simulink library "CalculationGallon"  (R2017b)
settings: Solver=VariableStepAuto  StartTime=0.0  StopTime=10.0  RelTol=1e-3
undefined symbols (not defined in the file): DiscIntNeverNeededParam, Engine
libraries: simulink x3
settings Model: Creator=Lyu19  LastModifiedBy=Lyu19

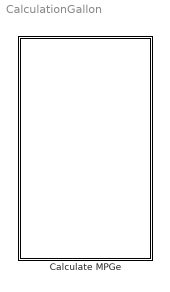
== system CalculationGallon ==
  Calculate MPGe : Subsystem

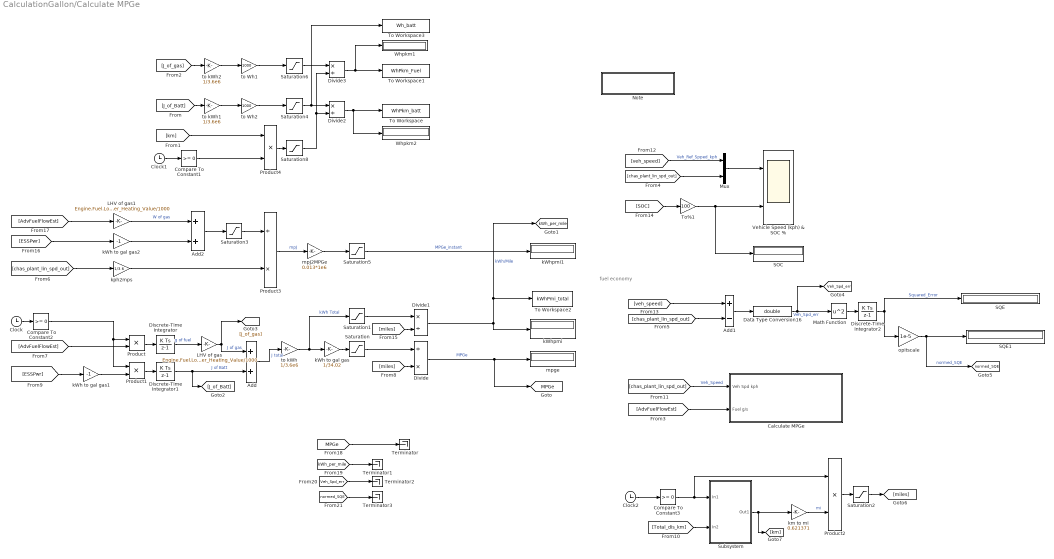
== system CalculationGallon/Calculate MPGe ==
  note: fuel economy
  Add : Sum
  Add1 : Sum  Inputs=+-
  Add2 : Sum
  Calculate MPGe : Subsystem
  Clock : Clock
  Clock1 : Clock
  Clock2 : Clock
  Compare To Constant1 : simulink/Logic and Bit Operations/Compare To Constant  relop=>=  const=0  OutDataTypeStr=boolean
  Compare To Constant2 : simulink/Logic and Bit Operations/Compare To Constant  relop=>=  const=0  OutDataTypeStr=boolean
  Compare To Constant3 : simulink/Logic and Bit Operations/Compare To Constant  relop=>=  const=0  OutDataTypeStr=boolean
  Data Type Conversion16 : DataTypeConversion  OutDataTypeStr=double
  Discrete-Time Integrator : DiscreteIntegrator  SampleTime=-1  ICPrevOutput=DiscIntNeverNeededParam  ICPrevScaledInput=DiscIntNeverNeededParam
  Discrete-Time Integrator1 : DiscreteIntegrator  SampleTime=-1  ICPrevOutput=DiscIntNeverNeededParam  ICPrevScaledInput=DiscIntNeverNeededParam
  Discrete-Time Integrator2 : DiscreteIntegrator  SampleTime=-1  ICPrevOutput=DiscIntNeverNeededParam  ICPrevScaledInput=DiscIntNeverNeededParam
  Divide : Product  Inputs=/*
  Divide1 : Product  Inputs=*/
  Divide2 : Product  Inputs=*/
  Divide3 : Product  Inputs=*/
  LHV of gas : Gain  Gain=Engine.Fuel.Lower_Heating_Value/1000
  LHV of gas1 : Gain  Gain=Engine.Fuel.Lower_Heating_Value/1000
  Math Function : Math  Operator=square  SaturateOnIntegerOverflow=on
  Mux : Mux  Inputs=2
  Note : Subsystem
  Product{,1..2,4} (4 alike) : Product
  Product3 : Product  Inputs=/*
  SOC : Display
  SQE : Display
  SQE1 : Display
  Saturation{,1..4,6,8} (7 alike) : Saturate  UpperLimit=inf  LowerLimit=1e-6
  Saturation5 : Saturate  UpperLimit=80  LowerLimit=1e-6
  Subsystem : Subsystem
  Terminator{,1..3} (4 alike) : Terminator
  To Workspace : ToWorkspace  VariableName=WhPkm_batt  SampleTime=-1
  To Workspace1 : ToWorkspace  VariableName=WhPkm_Fuel  SampleTime=-1
  To Workspace2 : ToWorkspace  VariableName=kWhPmi_total  SampleTime=-1
  To Workspace3 : ToWorkspace  VariableName=Wh_batt  SampleTime=-1
  To%1 : Gain  Gain=100
  Vehicle Speed (kph) & SOC % : Scope  NumInputPorts=2
  Whpkm1 : Display
  Whpkm2 : Display
  kWh to gal gas : Gain  Gain=1/34.02
  kWh to gal gas1 : Gain  Gain=-1
  kWh to gal gas2 : Gain  Gain=-1
  kWhpmi : Display
  kWhpmi1 : Display
  km to mi : Gain  Gain=0.621371
  kph2mps : Gain  Gain=1/3.6
  mpJ2MPGe : Gain  Gain=0.013*1e6
  mpge : Display
  opitscale : Gain  Gain=1e-5
  to Wh1 : Gain  Gain=1000
  to Wh2 : Gain  Gain=1000
  to kWh : Gain  Gain=1/3.6e6
  to kWh1 : Gain  Gain=1/3.6e6
  to kWh2 : Gain  Gain=1/3.6e6
  tag scope: MPGe=global, Veh_Spd_err=global, kWh_per_mile=global, normed_SQE=global
  wires:
  Discrete-Time Integrator/1 -> LHV of gas/1  "g of fuel"
  LHV of gas/1 -> Add/1, [J_of_gas]  "J of gas"
  Discrete-Time Integrator1/1 -> Add/2, [J_of_Batt]  "J of Batt"
  Add/1 -> to kWh/1  "J total"
  to kWh/1 -> kWh to gal gas/1, Saturation1/1  "kWh Total"
  km to mi/1 -> Product2/2  "mi"
  kWh to gal gas/1 -> Saturation/1
  Divide/1 -> [MPGe], mpge/1  "MPGe"
  [AdvFuelFlowEst] -> Product/2
  [Total_dis_km] -> Subsystem/2(In2)
  Saturation/1 -> Divide/1
  Saturation1/1 -> Divide1/1
  Divide1/1 -> kWhpmi/1, [kWh_per_mile], To Workspace2/1  "kWh/Mile"
  [veh_speed] -> Mux/1  "Veh_Ref_Spped_kph"
  Mux/1 -> Vehicle Speed (kph) & SOC %/1
  [chas_plant_lin_spd_out] -> Calculate MPGe/1(Veh Spd kph)  "Veh_Speed"
  Discrete-Time Integrator2/1 -> opitscale/1, SQE/1  "Squared_Error"
  Data Type Conversion16/1 -> Math Function/1, [Veh_Spd_err]  "Veh_Spd_err"
  opitscale/1 -> [normed_SQE], SQE1/1  "normed_SQE"
  Math Function/1 -> Discrete-Time Integrator2/1
  Saturation2/1 -> [miles]
  Subsystem/1(Out1) -> km to mi/1, [km]
  Clock/1 -> Compare To Constant2/1
  Product/1 -> Discrete-Time Integrator/1
  Compare To Constant2/1 -> Product1/1, Product/1
  Product1/1 -> Discrete-Time Integrator1/1
  Add1/1 -> Data Type Conversion16/1
  Product2/1 -> Saturation2/1
  LHV of gas1/1 -> Add2/1  "W of gas"
  Product3/1 -> mpJ2MPGe/1  "mpJ"
  mpJ2MPGe/1 -> Saturation5/1
  Add2/1 -> Saturation3/1
  Saturation5/1 -> kWhpmi1/1  "MPGe_instant"
  kph2mps/1 -> Product3/2
  Saturation3/1 -> Product3/1
  [J_of_Batt] -> to kWh1/1
  to kWh1/1 -> to Wh2/1
  to Wh2/1 -> Saturation4/1
  Saturation4/1 -> To Workspace3/1, Divide2/1
  Divide2/1 -> Whpkm2/1, To Workspace/1
  [J_of_gas] -> to kWh2/1
  to kWh2/1 -> to Wh1/1
  to Wh1/1 -> Saturation6/1
  Saturation6/1 -> Divide3/1
  Divide3/1 -> Whpkm1/1, To Workspace1/1
  [km] -> Product4/1
  Product4/1 -> Saturation8/1
  Saturation8/1 -> Divide3/2, Divide2/2
  [ESSPwr] -> kWh to gal gas1/1
  kWh to gal gas1/1 -> Product1/2
  Clock1/1 -> Compare To Constant1/1
  Compare To Constant1/1 -> Product4/2
  [AdvFuelFlowEst] -> Calculate MPGe/2(Fuel g/s)
  [chas_plant_lin_spd_out] -> Add1/2
  [chas_plant_lin_spd_out] -> Mux/2
  [chas_plant_lin_spd_out] -> kph2mps/1
  [veh_speed] -> Add1/1
  [SOC] -> To%1/1
  To%1/1 -> SOC/1, Vehicle Speed (kph) & SOC %/2
  Clock2/1 -> Compare To Constant3/1
  Compare To Constant3/1 -> Product2/1, Subsystem/1(In1)
  [miles] -> Divide/2
  [miles] -> Divide1/2
  [ESSPwr] -> kWh to gal gas2/1
  kWh to gal gas2/1 -> Add2/2
  [AdvFuelFlowEst] -> LHV of gas1/1
  [MPGe] -> Terminator/1
  [kWh_per_mile] -> Terminator1/1
  [Veh_Spd_err] -> Terminator2/1
  [normed_SQE] -> Terminator3/1

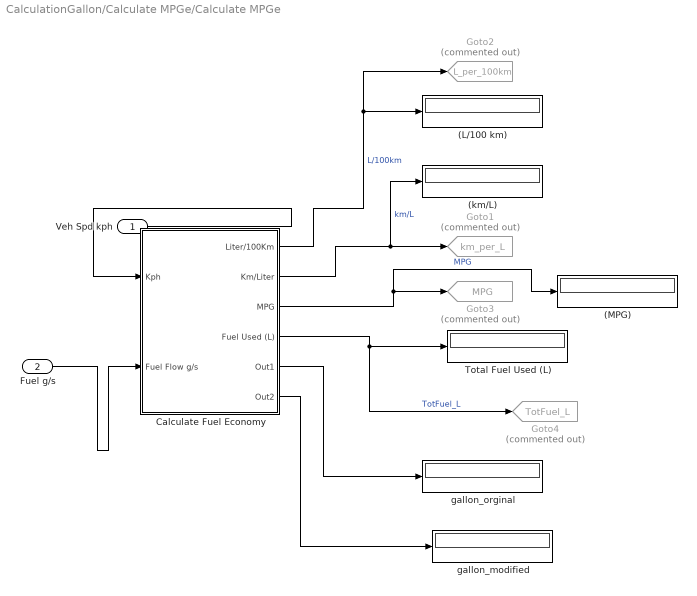
== system CalculationGallon/Calculate MPGe/Calculate MPGe ==
  Veh Spd kph : Inport
  Fuel g/s : Inport  Port=2
  (L/100 km) : Display
  (MPG) : Display
  (km/L) : Display
  Calculate Fuel Economy : Subsystem
  Goto1 : Goto  Commented=on  GotoTag=km_per_L  TagVisibility=global
  Goto2 : Goto  Commented=on  GotoTag=L_per_100km  TagVisibility=global
  Goto3 : Goto  Commented=on  GotoTag=MPG  TagVisibility=global
  Goto4 : Goto  Commented=on  GotoTag=TotFuel_L  TagVisibility=global
  Total Fuel Used (L) : Display
  gallon_modified : Display
  gallon_orginal : Display
  wires:
  Fuel g/s/1 -> Calculate Fuel Economy/2(Fuel Flow g/s)
  Calculate Fuel Economy/1(Liter/100Km) -> Goto2/1, (L/100 km)/1  "L/100km"
  Calculate Fuel Economy/3(MPG) -> Goto3/1, (MPG)/1  "MPG"
  Calculate Fuel Economy/4(Fuel Used (L)) -> Goto4/1, Total Fuel Used (L)/1  "TotFuel_L"
  Calculate Fuel Economy/2(Km/Liter) -> (km/L)/1, Goto1/1  "km/L"
  Veh Spd kph/1 -> Calculate Fuel Economy/1(Kph)
  Calculate Fuel Economy/5(Out1) -> gallon_orginal/1
  Calculate Fuel Economy/6(Out2) -> gallon_modified/1

== system CalculationGallon/Calculate MPGe/Note ==
  note: Note that this is calculating the
      | instantaneous MPGe over time
      | (includes fuel and battery energy used).
      |
      | You should also look at the SOC
      | or energy of the Battery at the end
      | of the cycle, and see what the delta
      | is between the start/end.  If more/less
      | energy is in the Battery at the end, you
      | should determine how you want to
      | account for this difference.  For example,
      | if you consider Plug-In capability to account
      | for energy used, you can factor the cost of
      | plugging in.
      | If you want to assume all energy for this
      | simulation should come from the energy
      | on board the vehicle, then you can make an
      | estimate of how much fuel you would need to
      | use to recharge the batteries using the engine
      | generator set.

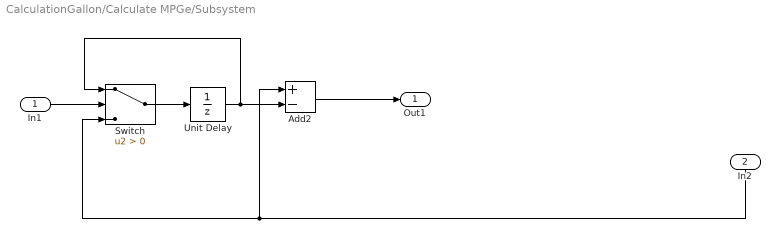
== system CalculationGallon/Calculate MPGe/Subsystem ==
  In1 : Inport
  In2 : Inport  Port=2
  Add2 : Sum  Inputs=+-
  Switch : Switch  Criteria=u2 > Threshold
  Unit Delay : UnitDelay  SampleTime=-1
  Out1 : Outport
  wires:
  Add2/1 -> Out1/1
  Unit Delay/1 -> Switch/1, Add2/2
  Switch/1 -> Unit Delay/1
  In1/1 -> Switch/2
  In2/1 -> Add2/1, Switch/3

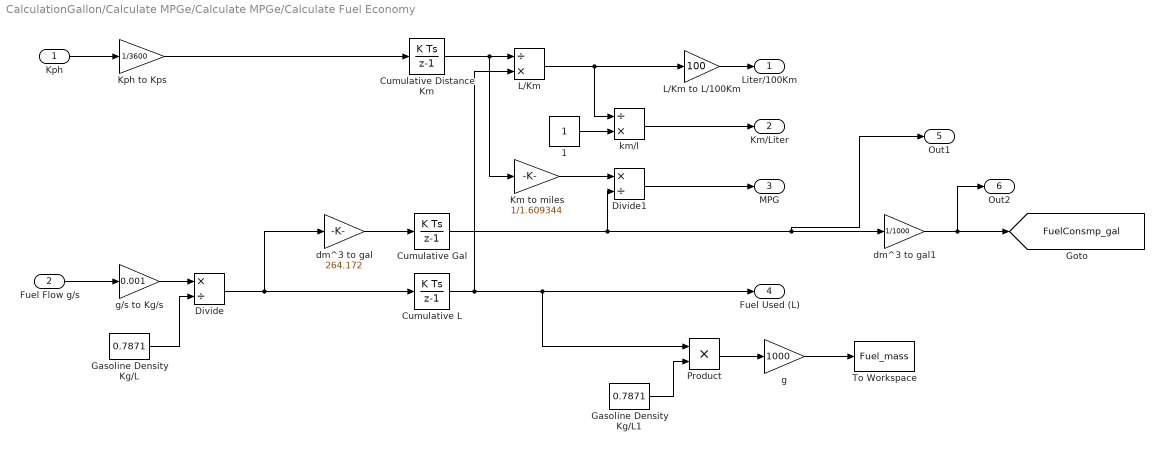
== system CalculationGallon/Calculate MPGe/Calculate MPGe/Calculate Fuel Economy ==
  Kph : Inport
  Fuel Flow g/s : Inport  Port=2
  1 : Constant
  Cumulative Distance Km : DiscreteIntegrator  InitialCondition=eps  SampleTime=-1  ICPrevOutput=DiscIntNeverNeededParam  ICPrevScaledInput=DiscIntNeverNeededParam
  Cumulative Gal : DiscreteIntegrator  InitialCondition=eps  SampleTime=-1  ICPrevOutput=DiscIntNeverNeededParam  ICPrevScaledInput=DiscIntNeverNeededParam
  Cumulative L : DiscreteIntegrator  InitialCondition=eps  SampleTime=-1  ICPrevOutput=DiscIntNeverNeededParam  ICPrevScaledInput=DiscIntNeverNeededParam
  Divide : Product  Inputs=*/
  Divide1 : Product  Inputs=*/
  Gasoline Density Kg/L : Constant  Value=0.7871
  Gasoline Density Kg/L1 : Constant  Value=0.7871
  Km to miles : Gain  Gain=1/1.609344
  Kph to Kps : Gain  Gain=1/3600
  L/Km : Product  Inputs=/*
  L/Km to L/100Km : Gain  Gain=100
  Product : Product
  To Workspace : ToWorkspace  VariableName=Fuel_mass  SampleTime=-1
  dm^3 to gal : Gain  Gain=264.172
  dm^3 to gal1 : Gain  Gain=1/1000
  g : Gain  Gain=1000
  g/s to Kg/s : Gain  Gain=0.001
  km/l : Product  Inputs=/*
  Liter/100Km : Outport
  Km/Liter : Outport  Port=2
  MPG : Outport  Port=3
  Fuel Used (L) : Outport  Port=4
  Out1 : Outport  Port=5
  Out2 : Outport  Port=6
  tag scope: FuelConsmp_gal=global
  wires:
  km/l/1 -> Km/Liter/1
  1/1 -> km/l/2
  Divide1/1 -> MPG/1
  L/Km to L/100Km/1 -> Liter/100Km/1
  Fuel Flow g/s/1 -> g/s to Kg/s/1
  Kph/1 -> Kph to Kps/1
  Cumulative Gal/1 -> Out1/1, dm^3 to gal1/1, Divide1/2
  Km to miles/1 -> Divide1/1
  L/Km/1 -> km/l/1, L/Km to L/100Km/1
  Cumulative Distance Km/1 -> Km to miles/1, L/Km/1
  Kph to Kps/1 -> Cumulative Distance Km/1
  dm^3 to gal/1 -> Cumulative Gal/1
  Divide/1 -> Cumulative L/1, dm^3 to gal/1
  Gasoline Density Kg/L/1 -> Divide/2
  g/s to Kg/s/1 -> Divide/1
  Cumulative L/1 -> L/Km/2, Product/1, Fuel Used (L)/1
  Gasoline Density Kg/L1/1 -> Product/2
  Product/1 -> g/1
  g/1 -> To Workspace/1
  dm^3 to gal1/1 -> Out2/1, [FuelConsmp_gal]
